simulink model "CM690A_HwAg0Meas"  (R2013b)
settings: Solver=FixedStepDiscrete  SolverMode=SingleTasking  StartTime=0.0  StopTime=22  FixedStep=0.002  RelTol=1e-3
undefined symbols (not defined in the file): ELECGLBPRM_DEGPERREV_DEGPERREV_F32, ELECGLBPRM_HWAGCENTROFFS_HWDEG_F32, ELECGLBPRM_HWAGSATNLOWRLIM_HWDEG_F32, ELECGLBPRM_HWAGSATNUPPRLIM_HWDEG_F32, ELECGLBPRM_HWAGSCA_ULS_F32, ELECGLBPRM_HWAGSPURGEARRAT_ULS_F32, ELECGLBPRM_HWAGSPURTORINGGEARRATSNSR0_ULS_F32, ELECGLBPRM_HWAGSPURTORINGGEARRATSNSR1_ULS_F32, ELECGLBPRM_NOFLT_CNT_U08, ELECGLBPRM_OFFSTRIMNOTPRFMD_CNT_U08, ELECGLBPRM_PRTCLFLT_CNT_U08, ELECGLBPRM_SKIPSTEPFLT_CNT_U08, ELECGLBPRM_SNSRINTFLT_CNT_U08, ELECGLBPRM_VRNRERRFLT_CNT_U08, FLTINJ_HWAG0MEAS_HWAG0, FLTINJ_HWAG0MEAS_TESTOK, HwAg0IfFlt, HwAg0MeasHwAg0IfFltFailStep, HwAg0MeasHwAg0IfFltPassStep, HwAg0MeasHwAg0Snsr0PrtclFltFailStep, HwAg0MeasHwAg0Snsr0PrtclFltPassStep, HwAg0MeasHwAg0Snsr1PrtclFltFailStep, HwAg0MeasHwAg0Snsr1PrtclFltPassStep, HwAg0MeasSnsr0Rev, HwAg0MeasSnsr1Rev, HwAg0MeasStep, HwAg0MeasVrnrErrThd, HwAg0MfgFlt, HwAg0Snsr0PrtclFlt, HwAg0Snsr1PrtclFlt, HWAG10THTOOTHTRIG_CNT_U08, HWAG11THTOOTHTRIG_CNT_U08, NtcSts1, sigbuilder_block, SigQlfr1
libraries: simulink x30, NxtrNvM x3
(part 5 of 5)

== system CM690A_HwAg0Meas/HwAg0Meas/HwAg0MeasPer2/Snsr0Read/RawHwAgRead/NewMsg/NoStsFlt/TestPass ==
  Snsr0Id : Inport
  Snsr0Data : Inport  Port=2
  Action Port : ActionPort  ActionType=then
  Bus Creator : BusCreator  Inputs=3
  CopyRight2 : Subsystem  Description=|  mask(Copyright Information){none=on}
      | Copyright info block.                                               
      |                                                                     
      | Place copyright information at the top of every subsystem in design.
      mask prompts: none "No parameters"
      mask help: Place copyright information at the top of every subsystem in design.
      mask Display:
      | NxtrConf = 'Nexteer Confidential';
      | 
      | sys = bdroot; %handle for the current model ("system")
      | first = get_param(sys,'Created');
      | first = first(end-3:end);  %year is last four digits
      | 
      | last = get_param(sys,'LastModifiedDate');
      | if isempty(last)
      |     last = datestr(now,'yyyy');
      | else
      |     last = last(end-3:end);
      | end
      | 
      | if strcmp(first,last)
      |     fprintf('%s -- Copyright %s Nexteer',NxtrConf,first)
      | else
      |     fprintf('%s -- %s%s- %s Nexteer',NxtrConf,char(169),first,last)
      | end
  If Action Subsystem : Subsystem  RequirementInfo={'linktype_rmi_doors' '0000cf45 (/ESG Group/FDD Module Requirements/EA4 Specific/CM690A_HwAg0Meas)' '#CM690A_49' 'true' 'REQ: CM690A_49' '' } %GIDa_6d19d2af_0719_4b38_a240_51d9758057ae  TreatAsAtomicUnit=on
  If Action Subsystem2 : Subsystem  RequirementInfo={'linktype_rmi_doors' '0000cf45 (/ESG Group/FDD Module Requirements/EA4 Specific/CM690A_HwAg0Meas)' '#CM690A_110' 'true' 'REQ: CM690A_110' '' } %GIDa_a044ca59_0b31_4dba_b68b_ab203ca2e6b5  TreatAsAtomicUnit=on
  If2 : If  IfExpression=u1 == 0
  Merge : Merge
  Merge1 : Merge
  Merge2 : Merge
  Out1 : Outport
  wires:
  Merge1/1 -> Bus Creator/2  "TestOk"
  Merge2/1 -> Bus Creator/3  "ParamByte"
  Merge/1 -> Bus Creator/1  "RawHwAg"
  Bus Creator/1 -> Out1/1
  Snsr0Id/1 -> If2/1
  If2/1 -> If Action Subsystem/Action
  If2/2 -> If Action Subsystem2/Action
  If Action Subsystem/1(RawHwAg) -> Merge/1
  If Action Subsystem2/1(RawHwAg) -> Merge/2
  If Action Subsystem/2(NtcSts) -> Merge1/1
  If Action Subsystem2/2(NtcSts) -> Merge1/2
  If Action Subsystem/3(ParamByte) -> Merge2/1
  If Action Subsystem2/3(ParamByte) -> Merge2/2
  Snsr0Data/1 -> If Action Subsystem/1(Snsr0Data)

== system CM690A_HwAg0Meas/HwAg0Meas/HwAg0MeasPer2/Snsr0Read/RawHwAgRead/NewMsg/STSFLT/CopyRight2 ==

== system CM690A_HwAg0Meas/HwAg0Meas/HwAg0MeasPer3/Snsr1Read/RawHwAgRead/NewMsg/NoStsFlt/CommFlt ==
  Action Port : ActionPort  ActionType=else
  Add : Sum
  Bus Creator1 : BusCreator  Inputs=3
  Constant : Constant  OutDataTypeStr=uint8
  CopyRight2 : Subsystem  Description=|  mask(Copyright Information){none=on}
      | Copyright info block.                                               
      |                                                                     
      | Place copyright information at the top of every subsystem in design.
      mask prompts: none "No parameters"
      mask help: Place copyright information at the top of every subsystem in design.
      mask Display:
      | NxtrConf = 'Nexteer Confidential';
      | 
      | sys = bdroot; %handle for the current model ("system")
      | first = get_param(sys,'Created');
      | first = first(end-3:end);  %year is last four digits
      | 
      | last = get_param(sys,'LastModifiedDate');
      | if isempty(last)
      |     last = datestr(now,'yyyy');
      | else
      |     last = last(end-3:end);
      | end
      | 
      | if strcmp(first,last)
      |     fprintf('%s -- Copyright %s Nexteer',NxtrConf,first)
      | else
      |     fprintf('%s -- %s%s- %s Nexteer',NxtrConf,char(169),first,last)
      | end
  Data Store Read : DataStoreRead  DataStoreName=HwAg0Snsr1IntSnsrErrCntr
  Data Store Write : DataStoreWrite  DataStoreName=HwAg0Snsr1IntSnsrErrCntr
  Data Type Conversion : DataTypeConversion  OutDataTypeStr=uint8
  Flt : Constant  Value=ELECGLBPRM_SNSRINTFLT_CNT_U08  OutDataTypeStr=uint8
  HwAg : Constant  Value=0  OutDataTypeStr=uint16
  NtcSts : simulink/Sources/Enumerated Constant  OutDataTypeStr=Enum: NtcSts1  Value=NtcSts1.NTCSTS_PREFAILD  SampleTime=inf
  Signal Conversion1 : SignalConversion
  Out2 : Outport
  wires:
  Flt/1 -> Bus Creator1/3  "ParamByte"
  NtcSts/1 -> Data Type Conversion/1
  HwAg/1 -> Bus Creator1/1  "RawHwAg"
  Bus Creator1/1 -> Signal Conversion1/1
  Signal Conversion1/1 -> Out2/1
  Data Type Conversion/1 -> Bus Creator1/2  "TestOk"
  Data Store Read/1 -> Add/1
  Constant/1 -> Add/2
  Add/1 -> Data Store Write/1

== system CM690A_HwAg0Meas/HwAg0Meas/HwAg0MeasPer3/Snsr1Read/RawHwAgRead/NewMsg/NoStsFlt/CopyRight2 ==

== system CM690A_HwAg0Meas/HwAg0Meas/HwAg0MeasPer3/Snsr1Read/RawHwAgRead/NewMsg/NoStsFlt/TestPass ==
  Snsr1Id : Inport
  Snsr1Data : Inport  Port=2
  Action Port : ActionPort  ActionType=then
  Bus Creator : BusCreator  Inputs=3
  CopyRight2 : Subsystem  Description=|  mask(Copyright Information){none=on}
      | Copyright info block.                                               
      |                                                                     
      | Place copyright information at the top of every subsystem in design.
      mask prompts: none "No parameters"
      mask help: Place copyright information at the top of every subsystem in design.
      mask Display:
      | NxtrConf = 'Nexteer Confidential';
      | 
      | sys = bdroot; %handle for the current model ("system")
      | first = get_param(sys,'Created');
      | first = first(end-3:end);  %year is last four digits
      | 
      | last = get_param(sys,'LastModifiedDate');
      | if isempty(last)
      |     last = datestr(now,'yyyy');
      | else
      |     last = last(end-3:end);
      | end
      | 
      | if strcmp(first,last)
      |     fprintf('%s -- Copyright %s Nexteer',NxtrConf,first)
      | else
      |     fprintf('%s -- %s%s- %s Nexteer',NxtrConf,char(169),first,last)
      | end
  If Action Subsystem : Subsystem  RequirementInfo={'linktype_rmi_doors' '0000cf45 (/ESG Group/FDD Module Requirements/EA4 Specific/CM690A_HwAg0Meas)' '#CM690A_67' 'true' 'REQ: CM690A_67' '' } %GIDa_f6f273d1_803e_441c_9b8d_aa660942fcf1  TreatAsAtomicUnit=on
  If Action Subsystem2 : Subsystem  RequirementInfo={'linktype_rmi_doors' '0000cf45 (/ESG Group/FDD Module Requirements/EA4 Specific/CM690A_HwAg0Meas)' '#CM690A_111' 'true' 'REQ: CM690A_111' '' } %GIDa_ba222b77_4f8c_464b_822e_140236467226  TreatAsAtomicUnit=on
  If2 : If  IfExpression=u1 == 1
  Merge : Merge
  Merge1 : Merge
  Merge2 : Merge
  Out1 : Outport
  wires:
  Merge1/1 -> Bus Creator/2  "TestOk"
  Merge2/1 -> Bus Creator/3  "ParamByte"
  Merge/1 -> Bus Creator/1  "RawHwAg"
  Bus Creator/1 -> Out1/1
  Snsr1Id/1 -> If2/1
  If2/1 -> If Action Subsystem/Action
  If2/2 -> If Action Subsystem2/Action
  If Action Subsystem/1(RawHwAg) -> Merge/1
  If Action Subsystem2/1(RawHwAg) -> Merge/2
  If Action Subsystem/2(NtcSts) -> Merge1/1
  If Action Subsystem2/2(NtcSts) -> Merge1/2
  If Action Subsystem/3(ParamByte) -> Merge2/1
  If Action Subsystem2/3(ParamByte) -> Merge2/2
  Snsr1Data/1 -> If Action Subsystem/1(Snsr1Data)

== system CM690A_HwAg0Meas/HwAg0Meas/HwAg0MeasPer3/Snsr1Read/RawHwAgRead/NewMsg/STSFLT/CopyRight2 ==

== system CM690A_HwAg0Meas/HwAg0Meas/HwAg0MeasPer4/HwAgRead/If Action Subsystem/AdjStepCalc/Diagc/CopyRight2 ==

== system CM690A_HwAg0Meas/HwAg0Meas/HwAg0MeasPer4/HwAgRead/If Action Subsystem/AdjStepCalc/Diagc/If Action  ==
  HwAg0Snsr0Rev : Inport
  HwAg0Snsr1Rev : Inport  Port=2
  HwAg0Snsr0Rel : Inport  Port=3
  HwAg0Snsr1Rel : Inport  Port=4
  HwAg0StepSeqNr : Inport  Port=5
  Action Port : ActionPort  ActionType=then
  AbsCalcHwAg0Snsr0 : Subsystem
  AbsCalcHwAg0Snsr1 : Subsystem
  CopyRight2 : Subsystem  Description=|  mask(Copyright Information){none=on}
      | Copyright info block.                                               
      |                                                                     
      | Place copyright information at the top of every subsystem in design.
      mask prompts: none "No parameters"
      mask help: Place copyright information at the top of every subsystem in design.
      mask Display:
      | NxtrConf = 'Nexteer Confidential';
      | 
      | sys = bdroot; %handle for the current model ("system")
      | first = get_param(sys,'Created');
      | first = first(end-3:end);  %year is last four digits
      | 
      | last = get_param(sys,'LastModifiedDate');
      | if isempty(last)
      |     last = datestr(now,'yyyy');
      | else
      |     last = last(end-3:end);
      | end
      | 
      | if strcmp(first,last)
      |     fprintf('%s -- Copyright %s Nexteer',NxtrConf,first)
      | else
      |     fprintf('%s -- %s%s- %s Nexteer',NxtrConf,char(169),first,last)
      | end
  PIM : DataStoreWrite  DataStoreName=HwAg0PrevStepSeqNr
  finalAbsAg : Subsystem
  HwAg0Meas : Outport
  HwAg0TestOk : Outport  Port=2
  ParamByte : Outport  Port=3
  wires:
  HwAg0Snsr0Rev/1 -> AbsCalcHwAg0Snsr0/2(HwAg0Snsr0Rev)
  AbsCalcHwAg0Snsr0/1(HwAg0Snsr0Abs) -> finalAbsAg/1(HwAg0Snsr0Abs)
  AbsCalcHwAg0Snsr1/1(HwAg0Snsr1Abs) -> finalAbsAg/2(HwAg0Snsr1Abs)
  finalAbsAg/1(HwAg0) -> HwAg0Meas/1
  finalAbsAg/2(TestOk) -> HwAg0TestOk/1
  finalAbsAg/3(ParamByte) -> ParamByte/1
  HwAg0Snsr0Rel/1 -> AbsCalcHwAg0Snsr0/1(HwAg0Snsr0Rel)
  HwAg0StepSeqNr/1 -> PIM/1
  HwAg0Snsr1Rel/1 -> AbsCalcHwAg0Snsr1/1(HwAg0Snsr1Rel)
  HwAg0Snsr1Rev/1 -> AbsCalcHwAg0Snsr1/2(HwAg0Snsr1Rev)

== system CM690A_HwAg0Meas/HwAg0Meas/HwAg0MeasPer4/HwAgRead/If Action Subsystem/AdjStepCalc/Diagc/If Action Skip ==
  Action Port : ActionPort  ActionType=else
  CopyRight2 : Subsystem  Description=|  mask(Copyright Information){none=on}
      | Copyright info block.                                               
      |                                                                     
      | Place copyright information at the top of every subsystem in design.
      mask prompts: none "No parameters"
      mask help: Place copyright information at the top of every subsystem in design.
      mask Display:
      | NxtrConf = 'Nexteer Confidential';
      | 
      | sys = bdroot; %handle for the current model ("system")
      | first = get_param(sys,'Created');
      | first = first(end-3:end);  %year is last four digits
      | 
      | last = get_param(sys,'LastModifiedDate');
      | if isempty(last)
      |     last = datestr(now,'yyyy');
      | else
      |     last = last(end-3:end);
      | end
      | 
      | if strcmp(first,last)
      |     fprintf('%s -- Copyright %s Nexteer',NxtrConf,first)
      | else
      |     fprintf('%s -- %s%s- %s Nexteer',NxtrConf,char(169),first,last)
      | end
  Data Type Conversion : DataTypeConversion  OutDataTypeStr=uint8
  Flt : Constant  Value=ELECGLBPRM_SKIPSTEPFLT_CNT_U08  OutDataTypeStr=uint8
  HwAg0 : Constant  Value=0  OutDataTypeStr=single
  NtcSts : simulink/Sources/Enumerated Constant  OutDataTypeStr=Enum: NtcSts1  Value=NtcSts1.NTCSTS_PREFAILD  SampleTime=inf
  HwAg0Meas : Outport
  HwAg0TestOk : Outport  Port=2  OutDataTypeStr=uint8
  ParamByte : Outport  Port=3
  wires:
  NtcSts/1 -> Data Type Conversion/1
  Flt/1 -> ParamByte/1
  HwAg0/1 -> HwAg0Meas/1
  Data Type Conversion/1 -> HwAg0TestOk/1

== system CM690A_HwAg0Meas/HwAg0Meas/HwAg0MeasPer4/HwAgRead/If Action Subsystem/AdjStepCalc/InitStep/CopyRight2 ==

== system CM690A_HwAg0Meas/HwAg0Meas/HwAg0MeasPer4/HwAgRead/If Action Subsystem/AdjStepCalc/InitStep/DoNothing ==
  Action Port : ActionPort  ActionType=else
  CopyRight2 : Subsystem  Description=|  mask(Copyright Information){none=on}
      | Copyright info block.                                               
      |                                                                     
      | Place copyright information at the top of every subsystem in design.
      mask prompts: none "No parameters"
      mask help: Place copyright information at the top of every subsystem in design.
      mask Display:
      | NxtrConf = 'Nexteer Confidential';
      | 
      | sys = bdroot; %handle for the current model ("system")
      | first = get_param(sys,'Created');
      | first = first(end-3:end);  %year is last four digits
      | 
      | last = get_param(sys,'LastModifiedDate');
      | if isempty(last)
      |     last = datestr(now,'yyyy');
      | else
      |     last = last(end-3:end);
      | end
      | 
      | if strcmp(first,last)
      |     fprintf('%s -- Copyright %s Nexteer',NxtrConf,first)
      | else
      |     fprintf('%s -- %s%s- %s Nexteer',NxtrConf,char(169),first,last)
      | end

== system CM690A_HwAg0Meas/HwAg0Meas/HwAg0MeasPer4/HwAgRead/If Action Subsystem/AdjStepCalc/InitStep/Else ==
  HwAg0StepSeqNr : Inport
  Action Port : ActionPort  ActionType=then
  Constant : Constant  OutDataTypeStr=boolean
  CopyRight2 : Subsystem  Description=|  mask(Copyright Information){none=on}
      | Copyright info block.                                               
      |                                                                     
      | Place copyright information at the top of every subsystem in design.
      mask prompts: none "No parameters"
      mask help: Place copyright information at the top of every subsystem in design.
      mask Display:
      | NxtrConf = 'Nexteer Confidential';
      | 
      | sys = bdroot; %handle for the current model ("system")
      | first = get_param(sys,'Created');
      | first = first(end-3:end);  %year is last four digits
      | 
      | last = get_param(sys,'LastModifiedDate');
      | if isempty(last)
      |     last = datestr(now,'yyyy');
      | else
      |     last = last(end-3:end);
      | end
      | 
      | if strcmp(first,last)
      |     fprintf('%s -- Copyright %s Nexteer',NxtrConf,first)
      | else
      |     fprintf('%s -- %s%s- %s Nexteer',NxtrConf,char(169),first,last)
      | end
  PIM : DataStoreWrite  DataStoreName=HwAg0PrevStepSeqNr
  PIM1 : DataStoreWrite  DataStoreName=HwAg0InitStepSeqNrCmpl
  wires:
  HwAg0StepSeqNr/1 -> PIM/1
  Constant/1 -> PIM1/1

== system CM690A_HwAg0Meas/HwAg0Meas/HwAg0MeasPer4/HwAgRead/If Action Subsystem/AdjStepCalc/Intpn/CopyRight2 ==

== system CM690A_HwAg0Meas/HwAg0Meas/HwAg0MeasPer4/HwAgRead/If Action Subsystem/AdjStepCalc/Intpn/StepCalc ==
  HwAg0Snsr0Rel : Inport
  HwAg0Snsr1Rel : Inport  Port=2
  Add : Sum  Inputs=+-
  CopyRight2 : Subsystem  Description=|  mask(Copyright Information){none=on}
      | Copyright info block.                                               
      |                                                                     
      | Place copyright information at the top of every subsystem in design.
      mask prompts: none "No parameters"
      mask help: Place copyright information at the top of every subsystem in design.
      mask Display:
      | NxtrConf = 'Nexteer Confidential';
      | 
      | sys = bdroot; %handle for the current model ("system")
      | first = get_param(sys,'Created');
      | first = first(end-3:end);  %year is last four digits
      | 
      | last = get_param(sys,'LastModifiedDate');
      | if isempty(last)
      |     last = datestr(now,'yyyy');
      | else
      |     last = last(end-3:end);
      | end
      | 
      | if strcmp(first,last)
      |     fprintf('%s -- Copyright %s Nexteer',NxtrConf,first)
      | else
      |     fprintf('%s -- %s%s- %s Nexteer',NxtrConf,char(169),first,last)
      | end
  Data Type Conversion1 : DataTypeConversion  OutDataTypeStr=single
  HwAgSpurGearRat : Constant  Value=ELECGLBPRM_HWAGSPURGEARRAT_ULS_F32  OutDataTypeStr=single
  Product : Product
  Scope : Scope  NumInputPorts=4
      settings: ShowLegends=on  TimeRange=10  YMin=0~0~0~-150  YMax=400~400~400~350  SaveName=ScopeData10
  HwAg0Step : Outport  OutDataTypeStr=single
  wires:
  Data Type Conversion1/1 -> Product/1
  Product/1 -> Add/2, Scope/3  "11thMultiplication"
  HwAgSpurGearRat/1 -> Product/2
  Add/1 -> Scope/4, HwAg0Step/1  "Step Val"
  HwAg0Snsr1Rel/1 -> Data Type Conversion1/1, Scope/2  "11ToothRel"
  HwAg0Snsr0Rel/1 -> Scope/1, Add/1  "10ToothRel"

== system CM690A_HwAg0Meas/HwAg0Meas/HwAg0MeasPer2/Snsr0Read/RawHwAgRead/NewMsg/NoStsFlt/CommFlt/CopyRight2 ==

== system CM690A_HwAg0Meas/HwAg0Meas/HwAg0MeasPer2/Snsr0Read/RawHwAgRead/NewMsg/NoStsFlt/TestPass/CopyRight2 ==

== system CM690A_HwAg0Meas/HwAg0Meas/HwAg0MeasPer2/Snsr0Read/RawHwAgRead/NewMsg/NoStsFlt/TestPass/If Action Subsystem ==
  note: Information only:
      |
      | - Correct Sensor As identified
  Snsr0Data : Inport
  Action Port : ActionPort  ActionType=then
  CopyRight2 : Subsystem  Description=|  mask(Copyright Information){none=on}
      | Copyright info block.                                               
      |                                                                     
      | Place copyright information at the top of every subsystem in design.
      mask prompts: none "No parameters"
      mask help: Place copyright information at the top of every subsystem in design.
      mask Display:
      | NxtrConf = 'Nexteer Confidential';
      | 
      | sys = bdroot; %handle for the current model ("system")
      | first = get_param(sys,'Created');
      | first = first(end-3:end);  %year is last four digits
      | 
      | last = get_param(sys,'LastModifiedDate');
      | if isempty(last)
      |     last = datestr(now,'yyyy');
      | else
      |     last = last(end-3:end);
      | end
      | 
      | if strcmp(first,last)
      |     fprintf('%s -- Copyright %s Nexteer',NxtrConf,first)
      | else
      |     fprintf('%s -- %s%s- %s Nexteer',NxtrConf,char(169),first,last)
      | end
  Data Type Conversion : DataTypeConversion  OutDataTypeStr=uint8
  NoFlt : Constant  RequirementInfo={} %GIDa_09607e89_3d4c_4382_a474_d3f95f867ac5  Value=ELECGLBPRM_NOFLT_CNT_U08  OutDataTypeStr=uint8
  NtcSts1 : simulink/Sources/Enumerated Constant  OutDataTypeStr=Enum: NtcSts1  Value=NtcSts1.NTCSTS_PREPASSD  SampleTime=inf
  RawHwAg : Outport
  NtcSts : Outport  Port=2
  ParamByte : Outport  Port=3
  wires:
  NtcSts1/1 -> Data Type Conversion/1
  Snsr0Data/1 -> RawHwAg/1
  NoFlt/1 -> ParamByte/1
  Data Type Conversion/1 -> NtcSts/1

== system CM690A_HwAg0Meas/HwAg0Meas/HwAg0MeasPer2/Snsr0Read/RawHwAgRead/NewMsg/NoStsFlt/TestPass/If Action Subsystem2 ==
  note: Information only:
      |
      | - Perform Diagnostic If not expected, Sensor is out of Sync
  Action Port : ActionPort  ActionType=else
  Add : Sum
  Constant : Constant  OutDataTypeStr=uint8
  CopyRight2 : Subsystem  Description=|  mask(Copyright Information){none=on}
      | Copyright info block.                                               
      |                                                                     
      | Place copyright information at the top of every subsystem in design.
      mask prompts: none "No parameters"
      mask help: Place copyright information at the top of every subsystem in design.
      mask Display:
      | NxtrConf = 'Nexteer Confidential';
      | 
      | sys = bdroot; %handle for the current model ("system")
      | first = get_param(sys,'Created');
      | first = first(end-3:end);  %year is last four digits
      | 
      | last = get_param(sys,'LastModifiedDate');
      | if isempty(last)
      |     last = datestr(now,'yyyy');
      | else
      |     last = last(end-3:end);
      | end
      | 
      | if strcmp(first,last)
      |     fprintf('%s -- Copyright %s Nexteer',NxtrConf,first)
      | else
      |     fprintf('%s -- %s%s- %s Nexteer',NxtrConf,char(169),first,last)
      | end
  Data Store Read : DataStoreRead  DataStoreName=HwAg0Snsr0IdErrCntr
  Data Store Write : DataStoreWrite  DataStoreName=HwAg0Snsr0IdErrCntr
  Data Type Conversion : DataTypeConversion  OutDataTypeStr=uint8
  HwAg : Constant  Value=0  OutDataTypeStr=uint16
  NtcSts1 : simulink/Sources/Enumerated Constant  OutDataTypeStr=Enum: NtcSts1  Value=NtcSts1.NTCSTS_PREFAILD  SampleTime=inf
  PRTCL_FAULT : Constant  Value=ELECGLBPRM_PRTCLFLT_CNT_U08  OutDataTypeStr=uint8
  RawHwAg : Outport
  NtcSts : Outport  Port=2
  ParamByte : Outport  Port=3
  wires:
  HwAg/1 -> RawHwAg/1
  NtcSts1/1 -> Data Type Conversion/1
  PRTCL_FAULT/1 -> ParamByte/1
  Data Type Conversion/1 -> NtcSts/1
  Data Store Read/1 -> Add/1
  Constant/1 -> Add/2
  Add/1 -> Data Store Write/1

== system CM690A_HwAg0Meas/HwAg0Meas/HwAg0MeasPer3/Snsr1Read/RawHwAgRead/NewMsg/NoStsFlt/CommFlt/CopyRight2 ==

== system CM690A_HwAg0Meas/HwAg0Meas/HwAg0MeasPer3/Snsr1Read/RawHwAgRead/NewMsg/NoStsFlt/TestPass/CopyRight2 ==

== system CM690A_HwAg0Meas/HwAg0Meas/HwAg0MeasPer3/Snsr1Read/RawHwAgRead/NewMsg/NoStsFlt/TestPass/If Action Subsystem ==
  note: Information only:
      |
      | - Correct Sensor As identified
  Snsr1Data : Inport
  Action Port : ActionPort  ActionType=then
  CopyRight2 : Subsystem  Description=|  mask(Copyright Information){none=on}
      | Copyright info block.                                               
      |                                                                     
      | Place copyright information at the top of every subsystem in design.
      mask prompts: none "No parameters"
      mask help: Place copyright information at the top of every subsystem in design.
      mask Display:
      | NxtrConf = 'Nexteer Confidential';
      | 
      | sys = bdroot; %handle for the current model ("system")
      | first = get_param(sys,'Created');
      | first = first(end-3:end);  %year is last four digits
      | 
      | last = get_param(sys,'LastModifiedDate');
      | if isempty(last)
      |     last = datestr(now,'yyyy');
      | else
      |     last = last(end-3:end);
      | end
      | 
      | if strcmp(first,last)
      |     fprintf('%s -- Copyright %s Nexteer',NxtrConf,first)
      | else
      |     fprintf('%s -- %s%s- %s Nexteer',NxtrConf,char(169),first,last)
      | end
  Data Type Conversion : DataTypeConversion  OutDataTypeStr=uint8
  NoFlt : Constant  RequirementInfo={} %GIDa_e0d2f201_318b_4149_ba4d_e1c5536708fc  Value=ELECGLBPRM_NOFLT_CNT_U08  OutDataTypeStr=uint8
  NtcSts1 : simulink/Sources/Enumerated Constant  OutDataTypeStr=Enum: NtcSts1  Value=NtcSts1.NTCSTS_PREPASSD  SampleTime=inf
  RawHwAg : Outport
  NtcSts : Outport  Port=2
  ParamByte : Outport  Port=3
  wires:
  NtcSts1/1 -> Data Type Conversion/1
  NoFlt/1 -> ParamByte/1
  Data Type Conversion/1 -> NtcSts/1
  Snsr1Data/1 -> RawHwAg/1

== system CM690A_HwAg0Meas/HwAg0Meas/HwAg0MeasPer3/Snsr1Read/RawHwAgRead/NewMsg/NoStsFlt/TestPass/If Action Subsystem2 ==
  note: Information Purpose Only :
      |
      | Sensor Sending Message Out of Order or 11th Tooth Sensor not Responding
  Action Port : ActionPort  ActionType=else
  Add : Sum
  Constant : Constant  OutDataTypeStr=uint8
  CopyRight2 : Subsystem  Description=|  mask(Copyright Information){none=on}
      | Copyright info block.                                               
      |                                                                     
      | Place copyright information at the top of every subsystem in design.
      mask prompts: none "No parameters"
      mask help: Place copyright information at the top of every subsystem in design.
      mask Display:
      | NxtrConf = 'Nexteer Confidential';
      | 
      | sys = bdroot; %handle for the current model ("system")
      | first = get_param(sys,'Created');
      | first = first(end-3:end);  %year is last four digits
      | 
      | last = get_param(sys,'LastModifiedDate');
      | if isempty(last)
      |     last = datestr(now,'yyyy');
      | else
      |     last = last(end-3:end);
      | end
      | 
      | if strcmp(first,last)
      |     fprintf('%s -- Copyright %s Nexteer',NxtrConf,first)
      | else
      |     fprintf('%s -- %s%s- %s Nexteer',NxtrConf,char(169),first,last)
      | end
  Data Store Read : DataStoreRead  DataStoreName=HwAg0Snsr1IdErrCntr
  Data Store Write : DataStoreWrite  DataStoreName=HwAg0Snsr1IdErrCntr
  Data Type Conversion : DataTypeConversion  OutDataTypeStr=uint8
  HwAg : Constant  Value=0  OutDataTypeStr=uint16
  NtcSts1 : simulink/Sources/Enumerated Constant  OutDataTypeStr=Enum: NtcSts1  Value=NtcSts1.NTCSTS_PREFAILD  SampleTime=inf
  PRTCL_FAULT : Constant  Value=ELECGLBPRM_PRTCLFLT_CNT_U08  OutDataTypeStr=uint8
  RawHwAg : Outport
  NtcSts : Outport  Port=2
  ParamByte : Outport  Port=3
  wires:
  HwAg/1 -> RawHwAg/1
  NtcSts1/1 -> Data Type Conversion/1
  PRTCL_FAULT/1 -> ParamByte/1
  Data Type Conversion/1 -> NtcSts/1
  Data Store Read/1 -> Add/1
  Constant/1 -> Add/2
  Add/1 -> Data Store Write/1

== system CM690A_HwAg0Meas/HwAg0Meas/HwAg0MeasPer4/HwAgRead/If Action Subsystem/AdjStepCalc/Diagc/If Action /AbsCalcHwAg0Snsr0 ==
  HwAg0Snsr0Rel : Inport
  HwAg0Snsr0Rev : Inport  Port=2
  Add : Sum
  CopyRight2 : Subsystem  Description=|  mask(Copyright Information){none=on}
      | Copyright info block.                                               
      |                                                                     
      | Place copyright information at the top of every subsystem in design.
      mask prompts: none "No parameters"
      mask help: Place copyright information at the top of every subsystem in design.
      mask Display:
      | NxtrConf = 'Nexteer Confidential';
      | 
      | sys = bdroot; %handle for the current model ("system")
      | first = get_param(sys,'Created');
      | first = first(end-3:end);  %year is last four digits
      | 
      | last = get_param(sys,'LastModifiedDate');
      | if isempty(last)
      |     last = datestr(now,'yyyy');
      | else
      |     last = last(end-3:end);
      | end
      | 
      | if strcmp(first,last)
      |     fprintf('%s -- Copyright %s Nexteer',NxtrConf,first)
      | else
      |     fprintf('%s -- %s%s- %s Nexteer',NxtrConf,char(169),first,last)
      | end
  HwAgRevDeg : Constant  Value=ELECGLBPRM_DEGPERREV_DEGPERREV_F32  OutDataTypeStr=single
  HwAgRevDeg1 : Constant  Value=ELECGLBPRM_HWAGSPURTORINGGEARRATSNSR0_ULS_F32  OutDataTypeStr=single
  PIM : DataStoreWrite  RequirementInfo={'linktype_rmi_doors' '0000cf45 (/ESG Group/FDD Module Requirements/EA4 Specific/CM690A_HwAg0Meas)' '#CM690A_91' 'true' 'REQ: CM690A_91' '' } %GIDa_f592a1a9_8111_4669_8b6a_8fb7bdd897ca  DataStoreName=dHwAg0MeasSnsr0Abs
  Product : Product
  Product1 : Product
  HwAg0Snsr0Abs : Outport  OutDataTypeStr=single
  wires:
  HwAg0Snsr0Rev/1 -> Product/1
  HwAgRevDeg/1 -> Product/2
  HwAg0Snsr0Rel/1 -> Add/1
  Product/1 -> Add/2
  Add/1 -> Product1/1
  HwAgRevDeg1/1 -> Product1/2
  Product1/1 -> PIM/1, HwAg0Snsr0Abs/1

== system CM690A_HwAg0Meas/HwAg0Meas/HwAg0MeasPer4/HwAgRead/If Action Subsystem/AdjStepCalc/Diagc/If Action /AbsCalcHwAg0Snsr1 ==
  HwAg0Snsr1Rel : Inport
  HwAg0Snsr1Rev : Inport  Port=2
  Add : Sum
  CopyRight2 : Subsystem  Description=|  mask(Copyright Information){none=on}
      | Copyright info block.                                               
      |                                                                     
      | Place copyright information at the top of every subsystem in design.
      mask prompts: none "No parameters"
      mask help: Place copyright information at the top of every subsystem in design.
      mask Display:
      | NxtrConf = 'Nexteer Confidential';
      | 
      | sys = bdroot; %handle for the current model ("system")
      | first = get_param(sys,'Created');
      | first = first(end-3:end);  %year is last four digits
      | 
      | last = get_param(sys,'LastModifiedDate');
      | if isempty(last)
      |     last = datestr(now,'yyyy');
      | else
      |     last = last(end-3:end);
      | end
      | 
      | if strcmp(first,last)
      |     fprintf('%s -- Copyright %s Nexteer',NxtrConf,first)
      | else
      |     fprintf('%s -- %s%s- %s Nexteer',NxtrConf,char(169),first,last)
      | end
  HwAgRevDeg : Constant  Value=ELECGLBPRM_DEGPERREV_DEGPERREV_F32  OutDataTypeStr=single
  HwAgRevDeg1 : Constant  Value=ELECGLBPRM_HWAGSPURTORINGGEARRATSNSR1_ULS_F32  OutDataTypeStr=single
  PIM : DataStoreWrite  RequirementInfo={'linktype_rmi_doors' '0000cf45 (/ESG Group/FDD Module Requirements/EA4 Specific/CM690A_HwAg0Meas)' '#CM690A_91' 'true' 'REQ: CM690A_91' '' } %GIDa_52de4b61_e269_46df_a896_4ef452a38029  DataStoreName=dHwAg0MeasSnsr1Abs
  Product : Product
  Product1 : Product
  HwAg0Snsr1Abs : Outport  OutDataTypeStr=single
  wires:
  HwAg0Snsr1Rev/1 -> Product/1
  HwAgRevDeg/1 -> Product/2
  HwAg0Snsr1Rel/1 -> Add/1
  Product/1 -> Add/2
  Add/1 -> Product1/1
  HwAgRevDeg1/1 -> Product1/2
  Product1/1 -> PIM/1, HwAg0Snsr1Abs/1

== system CM690A_HwAg0Meas/HwAg0Meas/HwAg0MeasPer4/HwAgRead/If Action Subsystem/AdjStepCalc/Diagc/If Action /CopyRight2 ==

== system CM690A_HwAg0Meas/HwAg0Meas/HwAg0MeasPer4/HwAgRead/If Action Subsystem/AdjStepCalc/Diagc/If Action /finalAbsAg ==
  HwAg0Snsr0Abs : Inport
  HwAg0Snsr1Abs : Inport  Port=2
  Abs : Abs
  Constant1 : Constant  Value=HwAg0MeasVrnrErrThd
  CopyRight2 : Subsystem  Description=|  mask(Copyright Information){none=on}
      | Copyright info block.                                               
      |                                                                     
      | Place copyright information at the top of every subsystem in design.
      mask prompts: none "No parameters"
      mask help: Place copyright information at the top of every subsystem in design.
      mask Display:
      | NxtrConf = 'Nexteer Confidential';
      | 
      | sys = bdroot; %handle for the current model ("system")
      | first = get_param(sys,'Created');
      | first = first(end-3:end);  %year is last four digits
      | 
      | last = get_param(sys,'LastModifiedDate');
      | if isempty(last)
      |     last = datestr(now,'yyyy');
      | else
      |     last = last(end-3:end);
      | end
      | 
      | if strcmp(first,last)
      |     fprintf('%s -- Copyright %s Nexteer',NxtrConf,first)
      | else
      |     fprintf('%s -- %s%s- %s Nexteer',NxtrConf,char(169),first,last)
      | end
  Data Type Conversion : DataTypeConversion  OutDataTypeStr=single
  If : If  NumInputs=2  IfExpression=u1 < u2
  If Action Subsystem : Subsystem  RequirementInfo={'linktype_rmi_doors' '0000cf45 (/ESG Group/FDD Module Requirements/EA4 Specific/CM690A_HwAg0Meas)' '#CM690A_85' 'true' 'REQ: CM690A_85' '' } %GIDa_cca15f29_c5cb_4de7_afc7_eb7f7e9160b6  TreatAsAtomicUnit=on
  If Action Subsystem1 : Subsystem  RequirementInfo={'linktype_rmi_doors' '0000cf45 (/ESG Group/FDD Module Requirements/EA4 Specific/CM690A_HwAg0Meas)' '#CM690A_76' 'true' 'REQ: CM690A_76' '' } %GIDa_13883830_3d0e_4d8b_84a5_ad4032d50ee7  TreatAsAtomicUnit=on
  Merge : Merge
  Merge1 : Merge
  Merge2 : Merge
  Scope3 : Scope  NumInputPorts=3
      settings: TimeRange=10  YMin=100~0~0  YMax=750~65000~65000  SaveName=ScopeData7
  Sub : Sum  Inputs=+-
  HwAg0 : Outport  OutDataTypeStr=single
  TestOk : Outport  Port=2  OutDataTypeStr=uint8
  ParamByte : Outport  Port=3  OutDataTypeStr=uint8
  wires:
  HwAg0Snsr0Abs/1 -> Scope3/1, If Action Subsystem/1(HwAg0Snsr0Abs), Sub/1  "10toothAbs"
  HwAg0Snsr1Abs/1 -> Scope3/2, If Action Subsystem/2(HwAg0Snsr1Abs), Sub/2  "11ToothAbs"
  Sub/1 -> Abs/1
  Abs/1 -> Scope3/3, If/1  "VernierAbs"
  Constant1/1 -> Data Type Conversion/1
  If/1 -> If Action Subsystem/Action
  If/2 -> If Action Subsystem1/Action
  If Action Subsystem1/2(HwAg0TestOk) -> Merge/2
  If Action Subsystem/2(HwAg0TestOk) -> Merge/1
  Merge/1 -> TestOk/1
  If Action Subsystem/1(HwAg0Meas) -> Merge1/1
  If Action Subsystem/3(ParamByte) -> Merge2/1
  If Action Subsystem1/1(HwAg0Meas) -> Merge1/2
  If Action Subsystem1/3(ParamByte) -> Merge2/2
  Merge2/1 -> ParamByte/1
  Merge1/1 -> HwAg0/1
  Data Type Conversion/1 -> If/2

== system CM690A_HwAg0Meas/HwAg0Meas/HwAg0MeasPer4/HwAgRead/If Action Subsystem/AdjStepCalc/Diagc/If Action Skip/CopyRight2 ==

== system CM690A_HwAg0Meas/HwAg0Meas/HwAg0MeasPer4/HwAgRead/If Action Subsystem/AdjStepCalc/InitStep/DoNothing/CopyRight2 ==

== system CM690A_HwAg0Meas/HwAg0Meas/HwAg0MeasPer4/HwAgRead/If Action Subsystem/AdjStepCalc/InitStep/Else/CopyRight2 ==

== system CM690A_HwAg0Meas/HwAg0Meas/HwAg0MeasPer4/HwAgRead/If Action Subsystem/AdjStepCalc/Intpn/StepCalc/CopyRight2 ==

== system CM690A_HwAg0Meas/HwAg0Meas/HwAg0MeasPer2/Snsr0Read/RawHwAgRead/NewMsg/NoStsFlt/TestPass/If Action Subsystem/CopyRight2 ==

== system CM690A_HwAg0Meas/HwAg0Meas/HwAg0MeasPer2/Snsr0Read/RawHwAgRead/NewMsg/NoStsFlt/TestPass/If Action Subsystem2/CopyRight2 ==

== system CM690A_HwAg0Meas/HwAg0Meas/HwAg0MeasPer3/Snsr1Read/RawHwAgRead/NewMsg/NoStsFlt/TestPass/If Action Subsystem/CopyRight2 ==

== system CM690A_HwAg0Meas/HwAg0Meas/HwAg0MeasPer3/Snsr1Read/RawHwAgRead/NewMsg/NoStsFlt/TestPass/If Action Subsystem2/CopyRight2 ==

== system CM690A_HwAg0Meas/HwAg0Meas/HwAg0MeasPer4/HwAgRead/If Action Subsystem/AdjStepCalc/Diagc/If Action /AbsCalcHwAg0Snsr0/CopyRight2 ==

== system CM690A_HwAg0Meas/HwAg0Meas/HwAg0MeasPer4/HwAgRead/If Action Subsystem/AdjStepCalc/Diagc/If Action /AbsCalcHwAg0Snsr1/CopyRight2 ==

== system CM690A_HwAg0Meas/HwAg0Meas/HwAg0MeasPer4/HwAgRead/If Action Subsystem/AdjStepCalc/Diagc/If Action /finalAbsAg/CopyRight2 ==

== system CM690A_HwAg0Meas/HwAg0Meas/HwAg0MeasPer4/HwAgRead/If Action Subsystem/AdjStepCalc/Diagc/If Action /finalAbsAg/If Action Subsystem ==
  HwAg0Snsr0Abs : Inport
  HwAg0Snsr1Abs : Inport  Port=2
  Action Port : ActionPort  ActionType=then
  Add : Sum
  Add1 : Sum  Inputs=+-
  CopyRight2 : Subsystem  Description=|  mask(Copyright Information){none=on}
      | Copyright info block.                                               
      |                                                                     
      | Place copyright information at the top of every subsystem in design.
      mask prompts: none "No parameters"
      mask help: Place copyright information at the top of every subsystem in design.
      mask Display:
      | NxtrConf = 'Nexteer Confidential';
      | 
      | sys = bdroot; %handle for the current model ("system")
      | first = get_param(sys,'Created');
      | first = first(end-3:end);  %year is last four digits
      | 
      | last = get_param(sys,'LastModifiedDate');
      | if isempty(last)
      |     last = datestr(now,'yyyy');
      | else
      |     last = last(end-3:end);
      | end
      | 
      | if strcmp(first,last)
      |     fprintf('%s -- Copyright %s Nexteer',NxtrConf,first)
      | else
      |     fprintf('%s -- %s%s- %s Nexteer',NxtrConf,char(169),first,last)
      | end
  Data Type Conversion : DataTypeConversion  OutDataTypeStr=uint8
  NoFlt : Constant  RequirementInfo={} %GIDa_1a0bb186_0d6a_4e81_a950_611f3df4a586  Value=ELECGLBPRM_NOFLT_CNT_U08  OutDataTypeStr=uint8
  NoFlt1 : Constant  RequirementInfo={} %GIDa_e4852178_08c6_4328_94a7_b4ef9c71e826  Value=ELECGLBPRM_HWAGCENTROFFS_HWDEG_F32
  NtcSts : simulink/Sources/Enumerated Constant  OutDataTypeStr=Enum: NtcSts1  Value=NtcSts1.NTCSTS_PREPASSD  SampleTime=inf
  ShiftR : ArithShift  BitShiftNumber=1  BitShiftDirection=Right
  HwAg0Meas : Outport  OutDataTypeStr=single
  HwAg0TestOk : Outport  Port=2  OutDataTypeStr=uint8
  ParamByte : Outport  Port=3
  wires:
  Add/1 -> ShiftR/1
  ShiftR/1 -> Add1/1
  HwAg0Snsr0Abs/1 -> Add/1
  HwAg0Snsr1Abs/1 -> Add/2
  NoFlt/1 -> ParamByte/1
  NtcSts/1 -> Data Type Conversion/1
  Data Type Conversion/1 -> HwAg0TestOk/1
  NoFlt1/1 -> Add1/2
  Add1/1 -> HwAg0Meas/1

== system CM690A_HwAg0Meas/HwAg0Meas/HwAg0MeasPer4/HwAgRead/If Action Subsystem/AdjStepCalc/Diagc/If Action /finalAbsAg/If Action Subsystem1 ==
  Action Port : ActionPort  ActionType=else
  CopyRight2 : Subsystem  Description=|  mask(Copyright Information){none=on}
      | Copyright info block.                                               
      |                                                                     
      | Place copyright information at the top of every subsystem in design.
      mask prompts: none "No parameters"
      mask help: Place copyright information at the top of every subsystem in design.
      mask Display:
      | NxtrConf = 'Nexteer Confidential';
      | 
      | sys = bdroot; %handle for the current model ("system")
      | first = get_param(sys,'Created');
      | first = first(end-3:end);  %year is last four digits
      | 
      | last = get_param(sys,'LastModifiedDate');
      | if isempty(last)
      |     last = datestr(now,'yyyy');
      | else
      |     last = last(end-3:end);
      | end
      | 
      | if strcmp(first,last)
      |     fprintf('%s -- Copyright %s Nexteer',NxtrConf,first)
      | else
      |     fprintf('%s -- %s%s- %s Nexteer',NxtrConf,char(169),first,last)
      | end
  Data Type Conversion : DataTypeConversion  OutDataTypeStr=uint8
  Flt : Constant  Value=ELECGLBPRM_VRNRERRFLT_CNT_U08
  HwAg0 : Constant  Value=0  OutDataTypeStr=single
  NtcSts : simulink/Sources/Enumerated Constant  OutDataTypeStr=Enum: NtcSts1  Value=NtcSts1.NTCSTS_PREFAILD  SampleTime=inf
  HwAg0Meas : Outport
  HwAg0TestOk : Outport  Port=2  OutDataTypeStr=uint8
  ParamByte : Outport  Port=3  OutDataTypeStr=uint8
  wires:
  NtcSts/1 -> Data Type Conversion/1
  Flt/1 -> ParamByte/1
  HwAg0/1 -> HwAg0Meas/1
  Data Type Conversion/1 -> HwAg0TestOk/1

== system CM690A_HwAg0Meas/HwAg0Meas/HwAg0MeasPer4/HwAgRead/If Action Subsystem/AdjStepCalc/Diagc/If Action /finalAbsAg/If Action Subsystem/CopyRight2 ==

== system CM690A_HwAg0Meas/HwAg0Meas/HwAg0MeasPer4/HwAgRead/If Action Subsystem/AdjStepCalc/Diagc/If Action /finalAbsAg/If Action Subsystem1/CopyRight2 ==

== stateflow chart CM690A_HwAg0Meas/HwAg0Meas/HwAg0MeasPer4/HwAgRead/RollCnt ==
  settings: stateMachineType=MEALY_MACHINE
  (default) -> (junction 89) : {HwAg0RollgCntr = HwAg0MeasPrevRollCnt;}
  (junction 89) -> (junction 169) [order 1] : [ (TestOk ==2) || (TestOk ==0) ]
  (junction 89) -> (junction 93) [order 2] : {
      | HwAg0RollgCntr = HwAg0RollgCntr;
      | }
  (junction 169) -> (junction 93) [order 2] : {HwAg0RollgCntr = 0;}
  (junction 169) -> (junction 93) [order 1] : [(HwAg0RollgCntr+1) <= 255]
      | {HwAg0RollgCntr = HwAg0RollgCntr + 1;}
  (junction 93) -> (junction 188)
  data: HwAg0RollgCntr output uint8; TestOk input uint8; HwAg0MeasPrevRollCnt input uint8

== stateflow chart CM690A_HwAg0Meas/HwAg0Meas/HwAg0MeasPer4/HwAgRead/If Action Subsystem/SetNtcSts/ISO Fault Debounce Design ==
  settings: stateMachineType=MEALY_MACHINE
  note: NTCSTS_PASSD           (0)
      | NTCSTS_FAILD             (1)
      | NTCSTS_PREPASSD   (2)
      | NTCSTS_PREFAILD     (3)
      |
      | SIGQLFR_NORES        (0)
      | SIGQLFR_PASSD         (1)
      | SIGQLFR_FAILD           (2)
  note: Pass Loop
  note: Fail Loop
  note: 
  (default) -> (junction 89)
  (junction 89) -> (junction 95) [order 1] : [NtcSts ==3]
  (junction 89) -> (junction 93) [order 2] : [NtcSts ==2]
  (junction 89) -> (junction 141) [order 3] : [NtcSts ==1]
      | { ErrAcc = 32767;
      | Qualifier =2;
      |  }
  (junction 89) -> (junction 141) [order 4] : [NtcSts ==0]
      | { ErrAcc = -32768;
      | Qualifier=1;
      | }
  (junction 95) -> (junction 103) [order 2]
  (junction 95) -> (junction 111) [order 1] : [ErrAcc <=0]
      | {ErrAcc = DebStep;}
  (junction 93) -> (junction 123) [order 2] : {
      | ErrAcc = ErrAcc - DebStep;
      | }
  (junction 93) -> (junction 123) [order 1] : [(ErrAcc - DebStep) <= -32768]
      | { ErrAcc = -32768;
      | Qualifier=1;
      | }
  (junction 103) -> (junction 111) [order 1] : [(ErrAcc + DebStep) <32767]
      | {ErrAcc = ErrAcc + DebStep;}
  (junction 103) -> (junction 111) [order 2] : {ErrAcc = 32767;
      | Qualifier =2;}
  (junction 123) -> (junction 141)
  (junction 111) -> (junction 141)
  (junction 141) -> (junction 159) [order 2] : {ErrAcc = 0;
      | Qualifier =0;
      | }
  (junction 141) -> (junction 159) [order 1] : [SvcClr ==0]
  data: NtcSts input uint8; Qualifier output uint8; DebStep input uint16; ErrAcc local single; SvcClr input

== stateflow chart CM690A_HwAg0Meas/HwAg0Meas/HwAg0MeasPer5/SetNtcSts/ISO Fault Debounce Design ==
  settings: stateMachineType=MEALY_MACHINE
  note: NTCSTS_PASSD           (0)
      | NTCSTS_FAILD             (1)
      | NTCSTS_PREPASSD   (2)
      | NTCSTS_PREFAILD     (3)
      |
      | SIGQLFR_NORES        (0)
      | SIGQLFR_PASSD         (1)
      | SIGQLFR_FAILD           (2)
  note: Pass Loop
  note: Fail Loop
  note: 
  (default) -> (junction 89)
  (junction 89) -> (junction 95) [order 1] : [NtcSts ==3]
  (junction 89) -> (junction 93) [order 2] : [NtcSts ==2]
  (junction 89) -> (junction 141) [order 3] : [NtcSts ==1]
      | { ErrAcc = 32767;
      | Qualifier =2;
      |  }
  (junction 89) -> (junction 141) [order 4] : [NtcSts ==0]
      | { ErrAcc = -32768;
      | Qualifier=1;
      | }
  (junction 95) -> (junction 103) [order 2]
  (junction 95) -> (junction 111) [order 1] : [ErrAcc <=0]
      | {ErrAcc = DebStep;}
  (junction 93) -> (junction 123) [order 2] : {
      | ErrAcc = ErrAcc - DebStep;
      | }
  (junction 93) -> (junction 123) [order 1] : [(ErrAcc - DebStep) <= -32768]
      | { ErrAcc = -32768;
      | Qualifier=1;
      | }
  (junction 103) -> (junction 111) [order 1] : [(ErrAcc + DebStep) <32767]
      | {ErrAcc = ErrAcc + DebStep;}
  (junction 103) -> (junction 111) [order 2] : {ErrAcc = 32767;
      | Qualifier =2;}
  (junction 123) -> (junction 141)
  (junction 111) -> (junction 141)
  (junction 141) -> (junction 159) [order 2] : {ErrAcc = 0;
      | Qualifier =0;
      | }
  (junction 141) -> (junction 159) [order 1] : [SvcClr ==0]
  data: NtcSts input uint8; Qualifier output uint8; DebStep input uint16; ErrAcc local single; SvcClr input
